simulink model "HDVSim_BEV_Truck"  (R2019b)
settings: Solver=ode3  StartTime=0.0  StopTime=inf  FixedStep=sample_time  MaxStep=0.1  RelTol=1e-3  EnableMultiTasking=on
model workspace (MAT data in the model file):
  Bat.SOC_start = 1
  Bat.Voltage = 800
  Bat.Useable_range = 0.8
  Bat.Charge_cycles = 3202.25561185
  Bat.Useable_capacity = 800
  Bat.Efficiency_power_electronics = 0.95
  Bat.Type = 1
  Electric_Truck = 1
  FuelCell.P_nom = 0
  Fueltype = 7
  Hybrid_Truck = 1
  IZ12 = 3600
  M_el = 1000
  SOC_T_EM_completely_available = 0.5
  SOC_addition = 0.4
  SOC_el = 0.8
  SOC_target = 0.85
  Sailing_without_drag_torque = 0
  TCO = TCO
  TCO.Ratio_Trailer_Truck = [1 1]
  TCO.Price_increase_repurchase = [3.5 3.5]
  TCO.Daily_working_time = 8
  TCO.Other_works_day = 0.5
  TCO.Gross_hourly_wage_driver = 13
  TCO.Operating_days_year = 240
  TCO.Annual_gross_wage_driver = 24960
  TCO.Personnel_factor = 1.3
  TCO.Annual_gross_wage_truck = 32448
  TCO.Social_costs_percent = 25.75
  TCO.Social_costs_EUR = 8355
  TCO.Back_up_driver = 0
  TCO.Fees_day = 12
  TCO.Fees_year = 2880
  TCO.Driver_costs_other = 0
  TCO.Driving_personnel_costs_total = 43683
  TCO.Diesel_price = 0.95
  TCO.Diesel_price_external = 1
  TCO.Adblue_price = 0.68
  TCO.CNG_price = 0.88
  TCO.LNG_price = 0.81
  TCO.Electricity_price = 0.12
  TCO.Hydrogen_price = 9
  TCO.Interest_current_asset = 8.4
  TCO.Interest_fixed_asset = 8.4
  TCO.Administrative_costs = 10.7
  TCO.Driving_distance = 0
  TCO.Ratio_toll_route = 75
  TCO.Loading_time_combination = 0.25
  TCO.Unloading_time_combination = 0.25
  TCO.Ratio_empty_trips = 0
  TCO.Operating_life = [6 12]
  TCO.Tire_mileage = [140000 170000]
  TCO.Ratio_inhouse_tanking_diesel = 75
  TCO.Lubricant_consumption = 1
  TCO.Adblue_consumption = 4
  TCO.Afa_time_dependent = [100 100]
  TCO.Afa_power_dependent = [0 0]
  TCO.Current_asset = [6000 1400]
  TCO.Insurance_vehicle = [0 0]
  TCO.Insurance_transport = 1000
  TCO.Communication = 600
  TCO.Repair_maintenance_care = [0.13 0.025]
  TCO.Current_assets_interest_bearing = 622
  TCO.Results = table
  TCO.Results.data = {{[]; []; []; []; []; []; []; []; []; []; []; []; []; []; []; []; []; []; []; []; []; []; []}, {[]; []; []; []; []; []; []; []; []; []; []; []; []; []; []; []; []; []; []; []; []; []; []}, {[]; []; []; []; []; []; []; []; []; []; []; []; []; []; []; []; []; []; []; []; []; []; []}, {'#cccccc'; '#9DFF00'; '#CEFF00'; '#FFFF00'; '#FFDF00'; '#FFB900'; '#FF9200'; '#FF5D00'; '#FF7F7F'; '#FF2900'; '#cccccc'; '#00FF85'; '#00FFC6'; '#00FFF2'; '#00FFFF'; '#00DBFF'; '#00B3FF'; '#0088FF'; '#cccccc'; '#B100FF'; '#FF00FF'; '#FF00C0'; '#FF0070'}, [0; 1; 1; 1; 1; 1; 1; 0; 1; 0; 0; 1; 1; 1; 1; 1; 1; 0; 0; 0; 1; 1; 0]}
  TCO.Results.ndims = 2
  TCO.Results.nrows = 23
  TCO.Results.rownames = {'Time_dependent_vehicle_costs'; 'Amortisation_time_dependent'; 'Current_assets_interest_bearing'; 'Fixed_assets_interest_bearing'; 'Taxes'; 'Insurance'; 'Communication'; 'Sum_vehicle_costs'; 'Driving_personnel_costs_total'; 'Sum_fix_costs'; 'Performance_related_vehicle_costs'; 'Amortisation_performance_related'; 'Fuel_costs'; 'Adblue_costs'; 'Repair_costs'; 'Lubricant_costs'; 'Tire_costs'; 'Sum_variable_costs'; 'Sum_costs'; 'Sum_fix_variable_costs'; 'Overhead_costs'; 'Toll_costs'; 'Total_costs'}
  TCO.Results.nvars = 5
  TCO.Results.varnames = {'Euro_Year', 'Euro_km', 'Percent', 'Cellcolor', 'Diagramm'}
  TCO.Results.props.useVariableNamesOriginal = 0
  TCO.Results.props.useDimensionNamesOriginal = 0
  TCO.Results.props.CustomProps = struct()
  TCO.Results.props.VariableCustomProps = struct()
  TCO.Results.props.versionSavedFrom = 4
  TCO.Results.props.minCompatibleVersion = 1
  TCO.Results.props.incompatibilityMsg = ''
  TCO.Results.props.VersionSavedFrom = 4
  TCO.Results.props.Description = ''
  TCO.Results.props.VariableNamesOriginal = {}
  TCO.Results.props.DimensionNames = {'Row', 'Variables'}
  TCO.Results.props.DimensionNamesOriginal = {}
  TCO.Results.props.UserData = []
  TCO.Results.props.VariableDescriptions = {}
  TCO.Results.props.VariableUnits = {}
  TCO.Results.props.VariableContinuity = {}
  TCO_Trailer = 1
  T_distance_LPS_down = 250
  T_distance_LPS_up = 250
  VSim.Display = 3
  VSim.Opt = 0
  VSim.v_t = [0 0 0 0 0 0 6.20410078977 13.0955619562 19.9830639689 26.8635610218 33.7348315113 40.5726013287 46.6919481688 50.4292373299 51.5990732528 55.4690950813 59.3274381556 63.1733217217 67.0059768235 70.7546293457 74.2808623311 77.6099839176 80.7667223894 83.4687787689 85.9844105019 87.7679000427 86.6050016922 86.7064046745 86.7114286994 86.7139311054 86.7163374998 86.7187109942 86.7210536154]
  Vehicle = 'empty'
  WPT.Voltage = 0
  WPT.P_max = 120
  WPT.expansion = 0.42
  WPT.eta = 0.92
  WPT.SOC_target = 1
  WPT.SOC_electric_only = 1
  acquisitionCosts = acquisitionCosts
  acquisitionCosts.KA_ZM = 361928.055317
  acquisitionCosts.KG = 3917.83103379
  acquisitionCosts.Getr_m = 135.266288088
  acquisitionCosts.KMot = 4672
  acquisitionCosts.KH = 179973.93
  acquisitionCosts.Hybrid = 1
  acquisitionCosts.Elektro = 1
  acquisitionCosts.Bat = 168200
  acquisitionCosts.Bat_type = 1
  acquisitionCosts.Bat_m = 5298.01324503
  acquisitionCosts.Bat_kWh = 800
  acquisitionCosts.Bat_VK_Pouch = 176
  acquisitionCosts.Bat_VK_Cyl = 210
  acquisitionCosts.Ratio_BEV2PHEV = 1
  acquisitionCosts.EM = 7717.5
  acquisitionCosts.EM_Type = 2
  acquisitionCosts.EM_P_max = 750
  acquisitionCosts.LE = 3375
  acquisitionCosts.FC = 0
  acquisitionCosts.P_FC = 0
  acquisitionCosts.KTFC_VK = 608
  acquisitionCosts.KA = 0
  acquisitionCosts.v_diesel = 0
  acquisitionCosts.v_cng = 0
  acquisitionCosts.v_lng = 0
  acquisitionCosts.m_h2 = 0
  acquisitionCosts.KT = 0
  acquisitionCosts.KTD = 0
  acquisitionCosts.KTCNG = 0
  acquisitionCosts.KTLNG = 0
  acquisitionCosts.KTFC = 0
  addition_for_critical_slope = 0.01
  ambient.gravity = 9.80665
  ambient.air_density = 1.1883
  ambient.friction_coeff = 0.8
  auxiliary_consumers.onBattery = 1
  auxiliary_consumers.power = 3500
  critical_altitude_difference = 50
  cycle.distance = [0 1 5 31 59 82 101 122 140 164 178 192 ... (10614 elements, 10614x1)]
  cycle.speed = [0 8.33333333333 8.33333333333 8.33333333333 8.33333333333 8.33333333333 8.33333333333 8.33333333333 8.33333333333 8.33333333333 8.33333333333 8.33333333333 ... (10614 elements, 10614x1)]
  cycle.slope = [0 0 0.0147 0.0305 0.0436 0.0483 0.0498 0.0479 0.0407 0.0324 0.0203 -0.0071 ... (10614 elements, 10614x1)]
  cycle.stop_time = [1 1 1 0 0 0 0 0 0 0 0 0 ... (10614 elements, 10614x1)]
  cycle.altitude = [0 0 0 0 0 0 0 0 0 0 0 0 ... (10614 elements, 10614x1)]
  cycle.stop_end = 15
  cycle.stop_start = 5
  cycle.speed_init = 1
  cycle.delta12 = [0 0 0 0 0 0 0 0 0 0 0 0 ... (10614 elements, 1x10614)]
  cycle.delta23 = [0 0 0 0 0 0 0 0 0 0 0 0 ... (10614 elements, 1x10614)]
  dcycle = 22
  distance_1_PPC = 175
  distance_2_PPC = 200
  distance_PPC_altitude_difference = 10000
  driver.controller_proportional_gain = 230000
  driver.controller_integral_gain = 3000
  driver.slew_rate_throttle_in = 2
  driver.slew_rate_throttle_out = -2
  driver.slew_rate_brake_in = 2
  driver.slew_rate_brake_out = -2
  em.P_max = 646.662302279
  em.M_max = 2040.65740249
  em.n_eck = 2525
  em.n_max = 4418
  em.speed = [0 27.786163522 55.572327044 83.358490566 111.144654088 138.93081761 166.716981132 194.503144654 222.289308176 250.075471698 277.86163522 305.647798742 ... (160 elements, 1x160)]
  em.trq = [2040.65740001 2040.65740051 2040.65740051 2040.65740211 2040.65740211 2040.65740249 2040.65740051 2040.65740051 2040.65740051 2040.65740051 2040.65740249 2040.65740051 ... (160 elements, 1x160)]
  em.Type = 2
  em.noEM = 2
  em.efficiency.characteristic_map = [0.001 0.001 0.001 0.001 0.001 0.001 0.001 0.001 0.001 0.001 0.001 0.001 ... (25600 elements, 160x160)]
  em.efficiency.speed = [0 27.786163522 55.572327044 83.358490566 111.144654088 138.93081761 166.716981132 194.503144654 222.289308176 250.075471698 277.86163522 305.647798742 ... (160 elements, 1x160)]
  em.efficiency.torque = [0 12.8343169968 25.6686339935 38.5029509903 51.3372679871 64.1715849838 77.0059019806 89.8402189773 102.674535974 115.508852971 128.343169968 141.177486964 ... (160 elements, 1x160)]
  em.shift_parameter.n_pref = 2398.75
  em.shift_parameter.n2 = 505
  em.shift_parameter.n6 = 3534.4
  em.fuel.co2_per_kwh = 504
  engine.M_max = 0
  engine.number = 4
  final_drive.ratio = 5
  final_drive.trq_eff = 0.98
  ifElectric = 1
  ifOptimized = 0
  look_ahead_PPC = 250
  max_distance = 100000
  name = 'HDVSim_BEV_Truck'
  preditiveCruiseControl = 0
  sample_time = 0.1
  tank.v_diesel = 0
  tank.v_lng = 0
  tank.v_cng = 0
  tank.m_h2 = 0
  tires.radius = 0.4465
  tires.roll_drag_coeff.total = 0.0043
  transmission.init_gear = 1
  transmission.shift_time = 1
  transmission.ratios = [1.7284 1]
  transmission.trq_eff = [0.96 0.99]
  transmission.lamda = [1.01169037498 1.00821410391]
  transmission.z = 2
  v_PPC_delta = 2.77777777778
  v_max_electrical_drive_only = 13.8888888889
  vehicle.long_truck = 0
  vehicle.payload = 19300
  vehicle.frontal_area = 10.2
  vehicle.air_drag_coeff = 0.53
  vehicle.Fx_max = 90221.18
  vehicle.F_brake_max = 309890.14
  vehicle.mass = 17056.2573109
  vehicleProperties = vehicleProperties
  vehicleProperties.CO2_EM_Range = 100
  vehicleProperties.a_0_80_Range = 54
  vehicleProperties.BOK_ak = 2.55
  vehicleProperties.BOK_Range = 4.65
  vehicleProperties.V_Rel_ak = 0.55
  vehicleProperties.V_Rel_Range = 0.35
  vehicleProperties.VWF_ak = 0.9
  vehicleProperties.VWF_Range = 7.2
  weights = weights
  weights.m_Gearbox = 135.266288088
  weights.m_Retarder = 82
  weights.m_Battery = 5298.01324503
  weights.m_EM = 833.333333333
  weights.m_PwrElectr = 69.4444444444
  weights.m_Charger = 15
  weights.m_Trailer = 5400
  weights.m_Total = 11656.2573109
  weights.m_Base = 5223.2
  weights.Electric = 1
  weights.Hybrid = 1
  weights.max_Payload = 23943.7426891
  weights.m_Max = 41000
  x = 1
values from neighbouring files (symbols this model uses):
  transmission = Transmission_gearing(15.86, 7, 0, 0, final_drive.ratio)    [Parameterizing.m]
undefined symbols (not defined in the file or in its folder): Ion, Lithium, prospective_cruise_control, Vorausschauender_Tempomat
libraries: simulink x21, powerlib x2, electricdrivelib x1
(part 1 of 3)
settings Model: Creator=Alexander Suessmann  LastModifiedBy=ubuntu
settings DataIOCC: SaveFormat=Array  SignalLoggingSaveFormat=ModelDataLogs  SaveOutput=off  SignalLogging=off  DSMLogging=off  ReturnWorkspaceOutputs=off  SignalLoggingName=datalog
settings OptimizationCC: ExpressionDepthLimit=2147483647  InitFltsAndDblsToZero=on  LifeSpan=inf
settings DebuggingCC: UnderspecifiedInitializationDetection=Classic  MergeDetectMultiDrivingBlocksExec=none  SolverPrmCheckMsg=warning  MultiTaskDSMMsg=warning  MultiTaskCondExecSysMsg=none  FcnCallInpInsideContextMsg=warning  AllowSymbolicDim=off  StateNameClashWarn=warning  SFUnexpectedBacktrackingDiag=warning  SFNoUnconditionalDefaultTransitionDiag=warning  SFExecutionAtInitializationDiag=none  UnderSpecifiedDimensionMsg=warning  ArithmeticOperatorsInVariantConditions=warning
settings HardwareCC: ProdBitPerPointer=32  ProdBitPerSizeT=32  ProdBitPerPtrDiffT=32  ProdLargestAtomicFloat=None  ProdIntDivRoundTo=Undefined  ProdEndianess=Unspecified  ProdWordSize=32  ProdHWDeviceType=32-bit Generic
settings ModelReferenceCC: PropagateSignalLabelsOutOfModel=off
settings SFSimCC: SimUseLocalCustomCode=off  CustomCodeUndefinedFunction=UseInterfaceOnly
settings RTWCC: RTWUseLocalCustomCode=off
settings CodeAppCC: StateflowObjectComments=on
settings GRTTargetCC: TargetLangStandard=C89/C90 (ANSI)  GeneratePreprocessorConditionals=Disable all  CombineOutputUpdateFcns=off  GRTInterface=on
settings ConfigComp: CovMetricSettings=dw  CovHtmlReporting=on  CovSaveCumulativeToWorkspaceVar=on  CovSaveSingleToWorkspaceVar=on  CovExternalEMLEnable=off  CovSFcnEnable=off
settings SimscapeCC: SimscapeNormalizeSystem=off

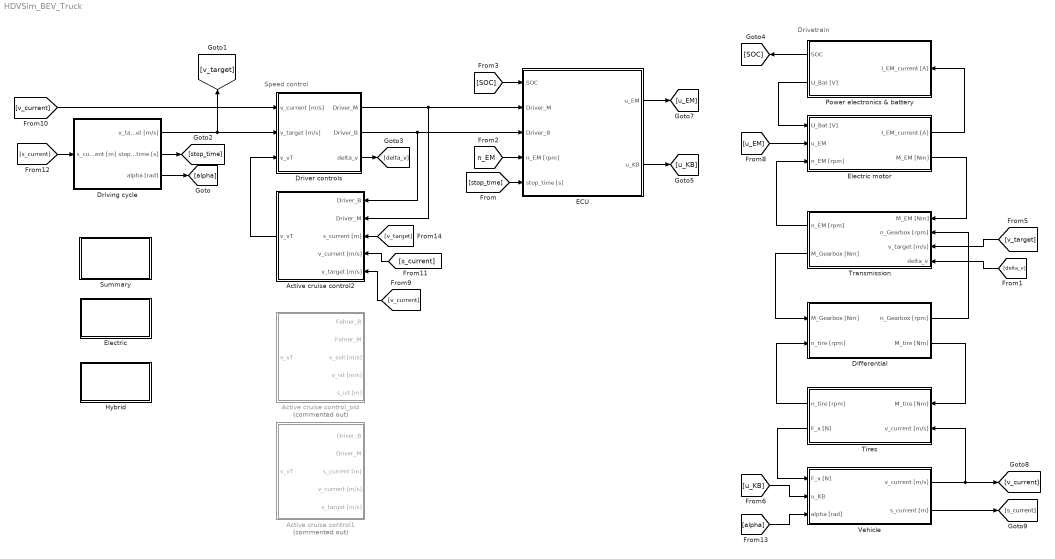
== system HDVSim_BEV_Truck ==
  note: Speed control
  note: Drivetrain
  Active cruise control1 : Subsystem  Commented=on
  Active cruise control2 : Subsystem
  Active cruise control_old : Subsystem  Commented=on
  Differential : Subsystem
  Driver controls : Subsystem
  Driving cycle : Subsystem
  ECU : Subsystem
  Electric : Subsystem
  Electric motor : Subsystem
  Hybrid : Subsystem
  Power electronics & battery : Subsystem
  Summary : Subsystem
  Tires : Subsystem
  Transmission : Subsystem
  Vehicle : Subsystem
  wires:
  Transmission/1(n_EM [rpm]) -> Electric motor/3(n_EM [rpm])
  Transmission/2(M_Gearbox [Nm]) -> Differential/1(M_Gearbox [Nm])
  Tires/1(n_tire [rpm]) -> Differential/2(n_tire [rpm])
  Differential/1(n_Gearbox [rpm]) -> Transmission/2(n_Gearbox [rpm])
  Differential/2(M_tire [Nm]) -> Tires/1(M_tire [Nm])
  Vehicle/1(v_current [m/s]) -> [v_current], Tires/2(v_current [m/s])
  Tires/2(F_x [N]) -> Vehicle/1(F_x [N])
  Driver controls/2(Driver_B) -> Active cruise control2/1(Driver_B), ECU/3(Driver_B)
  Electric motor/2(M_EM [Nm]) -> Transmission/1(M_EM [Nm])
  Electric motor/1(I_EM_current [A]) -> Power electronics & battery/1(I_EM_current [A])
  Power electronics & battery/2(U_Bat [V]) -> Electric motor/1(U_Bat [V])
  Active cruise control2/1(v_vT) -> Driver controls/3(v_vT)
  [n_EM] -> ECU/4(n_EM [rpm])
  Driving cycle/1(v_target [m/s]) -> [v_target], Driver controls/2(v_target [m/s])
  [v_current] -> Driver controls/1(v_current [m/s])
  [s_current] -> Driving cycle/1(s_current [m])
  Driver controls/1(Driver_M) -> Active cruise control2/2(Driver_M), ECU/2(Driver_M)
  Driving cycle/3(alpha [rad]) -> [alpha]
  Driving cycle/2(stop_time [s]) -> [stop_time]
  [stop_time] -> ECU/5(stop_time [s])
  Driver controls/3(delta_v) -> [delta_v]
  [SOC] -> ECU/1(SOC)
  [v_target] -> Active cruise control2/3(s_current [m])
  [s_current] -> Active cruise control2/4(v_current [m/s])
  [v_current] -> Active cruise control2/5(v_target [m/s])
  ECU/1(u_EM) -> [u_EM]
  ECU/2(u_KB) -> [u_KB]
  Power electronics & battery/1(SOC) -> [SOC]
  [u_EM] -> Electric motor/2(u_EM)
  [v_target] -> Transmission/3(v_target [m/s])
  [delta_v] -> Transmission/4(delta_v)
  Vehicle/2(s_current [m]) -> [s_current]
  [u_KB] -> Vehicle/2(u_KB)
  [alpha] -> Vehicle/3(alpha [rad])

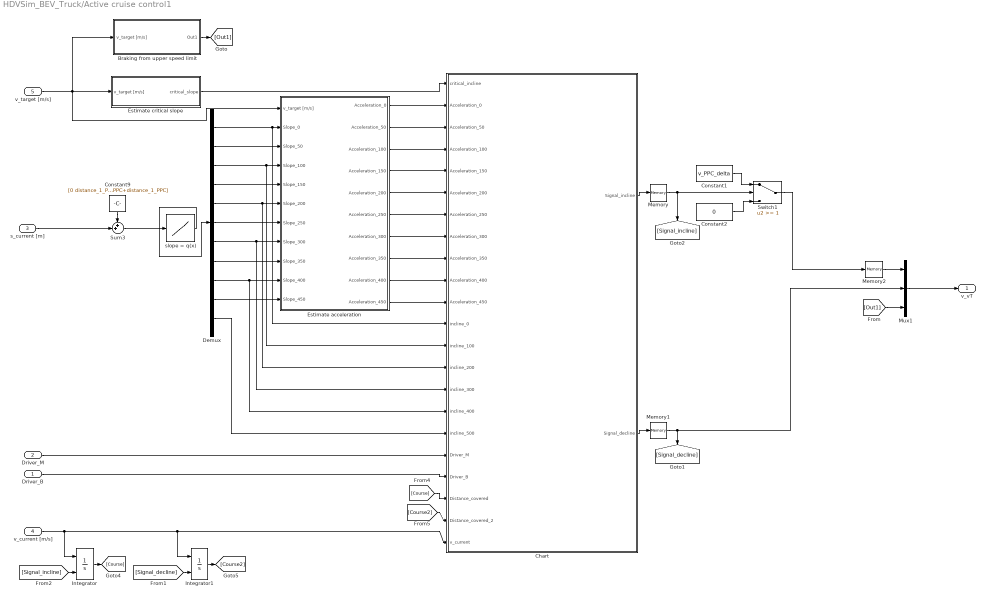
== system HDVSim_BEV_Truck/Active cruise control1 ==
  Driver_B : Inport
  Driver_M : Inport  Port=2
  s_current [m] : Inport  Port=3
  v_current [m/s] : Inport  Port=4
  v_target [m/s] : Inport  Port=5
  Braking from upper speed limit : Subsystem
  Chart : Stateflow chart  TreatAsAtomicUnit=on
  Constant1 : Constant  Value=v_PPC_delta
  Constant2 : Constant  Value=0
  Constant9 : Constant  Value=[0 distance_1_PPC/5 2*distance_1_PPC/5 3*distance_1_PPC/5 4*distance_1_PPC/5 distance_1_PPC 6*distance_1_PPC/5 7*distance_1_PPC/5 8*distance_1_PPC/5 9*distance_1_PPC/5 10*distance_1_PPC/5 look_ahead_PPC look_ahead_PPC+distance_1_PPC]
  Demux : Demux  Outputs=11
  Estimate acceleration : Subsystem
  Estimate critical slope : Subsystem
  Integrator : Integrator  ExternalReset=rising
  Integrator1 : Integrator  ExternalReset=rising
  Memory : Memory
  Memory1 : Memory
  Memory2 : Memory
  Mux1 : Mux  Inputs=3
  Sum3 : Sum  Inputs=++|
  Switch1 : Switch  Threshold=1
  slope = q(x) : Lookup  InputValues=cycle.distance  Table=cycle.slope  LookUpMeth=Interpolation-Use End Values
  v_vT : Outport  VectorParamsAs1DForOutWhenUnconnected=off
  wires:
  slope = q(x)/1 -> Demux/1
  Demux/1 -> Chart/12(incline_0), Estimate acceleration/2(Slope_0)
  Estimate critical slope/1(critical_slope) -> Chart/1(critical_incline)
  Chart/1(Signal_incline) -> Memory/1
  v_current [m/s]/1 -> Integrator/1, Integrator1/1, Chart/22(v_current)
  Memory/1 -> [Signal_incline], Switch1/2
  Mux1/1 -> v_vT/1
  Constant9/1 -> Sum3/1
  Sum3/1 -> slope = q(x)/1
  Estimate acceleration/1(Acceleration_0) -> Chart/2(Acceleration_0)
  Estimate acceleration/2(Acceleration_50) -> Chart/3(Acceleration_50)
  Estimate acceleration/3(Acceleration_100) -> Chart/4(Acceleration_100)
  Estimate acceleration/4(Acceleration_150) -> Chart/5(Acceleration_150)
  Estimate acceleration/5(Acceleration_200) -> Chart/6(Acceleration_200)
  Estimate acceleration/6(Acceleration_250) -> Chart/7(Acceleration_250)
  Estimate acceleration/7(Acceleration_300) -> Chart/8(Acceleration_300)
  Estimate acceleration/8(Acceleration_350) -> Chart/9(Acceleration_350)
  Chart/2(Signal_decline) -> Memory1/1
  Memory1/1 -> Mux1/2, [Signal_decline]
  Driver_B/1 -> Chart/19(Driver_B)
  Estimate acceleration/9(Acceleration_400) -> Chart/10(Acceleration_400)
  Estimate acceleration/10(Acceleration_450) -> Chart/11(Acceleration_450)
  Driver_M/1 -> Chart/18(Driver_M)
  Demux/2 -> Estimate acceleration/3(Slope_50)
  Demux/3 -> Chart/13(incline_100), Estimate acceleration/4(Slope_100)
  Demux/4 -> Estimate acceleration/5(Slope_150)
  Demux/5 -> Chart/14(incline_200), Estimate acceleration/6(Slope_200)
  Demux/6 -> Estimate acceleration/7("Slope_250 ")
  Demux/7 -> Chart/15(incline_300), Estimate acceleration/8(Slope_300)
  Demux/8 -> Estimate acceleration/9(Slope_350)
  Demux/9 -> Chart/16(incline_400), Estimate acceleration/10(Slope_400)
  Demux/10 -> Estimate acceleration/11(Slope_450)
  v_target [m/s]/1 -> Braking from upper speed limit/1(v_target [m/s]), Estimate acceleration/1(v_target [m/s]), Estimate critical slope/1(v_target [m/s])
  Memory2/1 -> Mux1/1
  Constant1/1 -> Switch1/1
  Constant2/1 -> Switch1/3
  Demux/11 -> Chart/17(incline_500)
  Switch1/1 -> Memory2/1
  s_current [m]/1 -> Sum3/2
  [Signal_decline] -> Integrator1/2
  Integrator1/1 -> [Course2]
  Integrator/1 -> [Course]
  [Signal_incline] -> Integrator/2
  [Course] -> Chart/20(Distance_covered)
  [Course2] -> Chart/21(Distance_covered_2)
  Braking from upper speed limit/1(Out1) -> [Out1]
  [Out1] -> Mux1/3

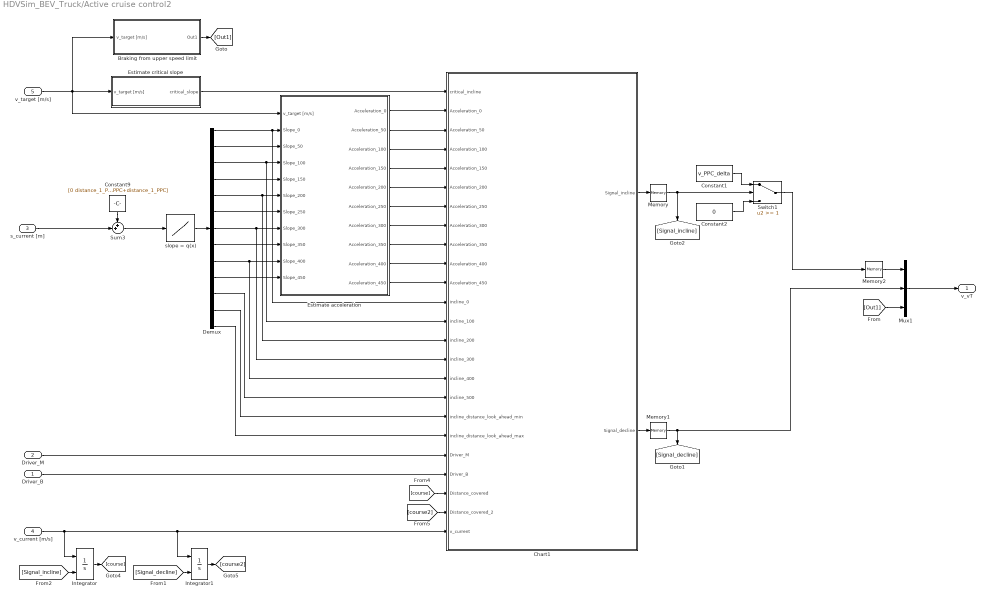
== system HDVSim_BEV_Truck/Active cruise control2 ==
  Driver_B : Inport
  Driver_M : Inport  Port=2
  s_current [m] : Inport  Port=3
  v_current [m/s] : Inport  Port=4
  v_target [m/s] : Inport  Port=5
  Braking from upper speed limit : Subsystem
  Chart1 : Stateflow chart  TreatAsAtomicUnit=on
  Constant1 : Constant  Value=v_PPC_delta
  Constant2 : Constant  Value=0
  Constant9 : Constant  Value=[0 distance_1_PPC/5 2*distance_1_PPC/5 3*distance_1_PPC/5 4*distance_1_PPC/5 distance_1_PPC 6*distance_1_PPC/5 7*distance_1_PPC/5 8*distance_1_PPC/5 9*distance_1_PPC/5 10*distance_1_PPC/5 look_ahead_PPC look_ahead_PPC+distance_1_PPC]
  Demux : Demux  Outputs=13
  Estimate acceleration : Subsystem
  Estimate critical slope : Subsystem
  Integrator : Integrator  ExternalReset=rising
  Integrator1 : Integrator  ExternalReset=rising
  Memory : Memory
  Memory1 : Memory
  Memory2 : Memory
  Mux1 : Mux  Inputs=3
  Sum3 : Sum  Inputs=++|
  Switch1 : Switch  Threshold=1
  slope = q(x) : Lookup  InputValues=cycle.distance  Table=cycle.slope  LookUpMeth=Interpolation-Use End Values
  v_vT : Outport  VectorParamsAs1DForOutWhenUnconnected=off
  wires:
  slope = q(x)/1 -> Demux/1
  Demux/1 -> Chart1/12(incline_0), Estimate acceleration/2(Slope_0)
  Estimate critical slope/1(critical_slope) -> Chart1/1(critical_incline)
  Chart1/1(Signal_incline) -> Memory/1
  v_current [m/s]/1 -> Integrator/1, Chart1/24(v_current), Integrator1/1
  Memory/1 -> [Signal_incline], Switch1/2
  Mux1/1 -> v_vT/1
  Constant9/1 -> Sum3/1
  Sum3/1 -> slope = q(x)/1
  Estimate acceleration/1(Acceleration_0) -> Chart1/2(Acceleration_0)
  Estimate acceleration/2(Acceleration_50) -> Chart1/3(Acceleration_50)
  Estimate acceleration/3(Acceleration_100) -> Chart1/4(Acceleration_100)
  Estimate acceleration/4(Acceleration_150) -> Chart1/5(Acceleration_150)
  Estimate acceleration/5(Acceleration_200) -> Chart1/6(Acceleration_200)
  Estimate acceleration/6(Acceleration_250) -> Chart1/7(Acceleration_250)
  Estimate acceleration/7(Acceleration_300) -> Chart1/8(Acceleration_300)
  Estimate acceleration/8(Acceleration_350) -> Chart1/9(Acceleration_350)
  Chart1/2(Signal_decline) -> Memory1/1
  Memory1/1 -> Mux1/2, [Signal_decline]
  Driver_B/1 -> Chart1/21(Driver_B)
  Estimate acceleration/9(Acceleration_400) -> Chart1/10(Acceleration_400)
  Estimate acceleration/10(Acceleration_450) -> Chart1/11(Acceleration_450)
  Driver_M/1 -> Chart1/20(Driver_M)
  Demux/2 -> Estimate acceleration/3(Slope_50)
  Demux/3 -> Chart1/13(incline_100), Estimate acceleration/4(Slope_100)
  Demux/4 -> Estimate acceleration/5(Slope_150)
  Demux/5 -> Chart1/14(incline_200), Estimate acceleration/6(Slope_200)
  Demux/6 -> Estimate acceleration/7("Slope_250 ")
  Demux/7 -> Chart1/15(incline_300), Estimate acceleration/8(Slope_300)
  Demux/8 -> Estimate acceleration/9(Slope_350)
  Demux/9 -> Chart1/16(incline_400), Estimate acceleration/10(Slope_400)
  Demux/10 -> Estimate acceleration/11(Slope_450)
  Demux/12 -> Chart1/18(incline_distance_look_ahead_min)
  Demux/13 -> Chart1/19(incline_distance_look_ahead_max)
  v_target [m/s]/1 -> Braking from upper speed limit/1(v_target [m/s]), Estimate acceleration/1(v_target [m/s]), Estimate critical slope/1(v_target [m/s])
  Memory2/1 -> Mux1/1
  Constant1/1 -> Switch1/1
  Constant2/1 -> Switch1/3
  Demux/11 -> Chart1/17(incline_500)
  Switch1/1 -> Memory2/1
  s_current [m]/1 -> Sum3/2
  [Signal_decline] -> Integrator1/2
  Integrator1/1 -> [course2]
  Integrator/1 -> [course]
  [Signal_incline] -> Integrator/2
  [course] -> Chart1/22(Distance_covered)
  [course2] -> Chart1/23(Distance_covered_2)
  Braking from upper speed limit/1(Out1) -> [Out1]
  [Out1] -> Mux1/3

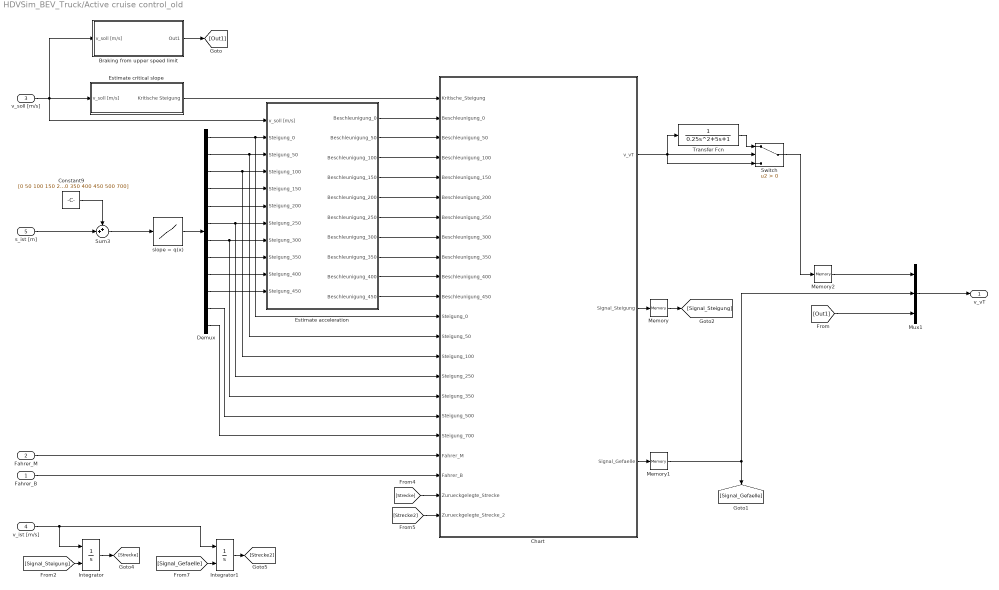
== system HDVSim_BEV_Truck/Active cruise control_old ==
  Fahrer_B : Inport
  Fahrer_M : Inport  Port=2
  v_soll [m/s] : Inport  Port=3
  v_ist [m/s] : Inport  Port=4
  s_ist [m] : Inport  Port=5
  Braking from upper speed limit : Subsystem
  Chart : Stateflow chart  TreatAsAtomicUnit=on
  Constant9 : Constant  Value=[0 50 100 150 200 250 300 350 400 450 500 700]
  Demux : Demux  Outputs=12
  Estimate acceleration : Subsystem
  Estimate critical slope : Subsystem
  Integrator : Integrator  ExternalReset=rising
  Integrator1 : Integrator  ExternalReset=rising
  Memory : Memory
  Memory1 : Memory
  Memory2 : Memory
  Mux1 : Mux  Inputs=3
  Sum3 : Sum  Inputs=++|
  Switch : Switch  Criteria=u2 > Threshold
  Transfer Fcn : TransferFcn  Denominator=[0.25 5 1]
  slope = q(x) : Lookup  InputValues=cycle.distance  Table=cycle.slope  LookUpMeth=Interpolation-Use End Values
  v_vT : Outport  VectorParamsAs1DForOutWhenUnconnected=off
  wires:
  slope = q(x)/1 -> Demux/1
  Demux/1 -> Estimate acceleration/2(Steigung_0), Chart/12(Steigung_0)
  Estimate critical slope/1(Kritische Steigung) -> Chart/1(Kritische_Steigung)
  Chart/2(Signal_Steigung) -> Memory/1
  Mux1/1 -> v_vT/1
  Constant9/1 -> Sum3/1
  s_ist [m]/1 -> Sum3/2
  Sum3/1 -> slope = q(x)/1
  Estimate acceleration/1(Beschleunigung_0) -> Chart/2(Beschleunigung_0)
  Estimate acceleration/2(Beschleunigung_50) -> Chart/3(Beschleunigung_50)
  Estimate acceleration/3(Beschleunigung_100) -> Chart/4(Beschleunigung_100)
  Estimate acceleration/4(Beschleunigung_150) -> Chart/5(Beschleunigung_150)
  Estimate acceleration/5(Beschleunigung_200) -> Chart/6(Beschleunigung_200)
  Estimate acceleration/6(Beschleunigung_250) -> Chart/7(Beschleunigung_250)
  Estimate acceleration/7(Beschleunigung_300) -> Chart/8(Beschleunigung_300)
  Estimate acceleration/8(Beschleunigung_350) -> Chart/9(Beschleunigung_350)
  Chart/3(Signal_Gefaelle) -> Memory1/1
  Memory1/1 -> [Signal_Gefaelle], Mux1/2
  Fahrer_B/1 -> Chart/20(Fahrer_B)
  Estimate acceleration/9(Beschleunigung_400) -> Chart/10(Beschleunigung_400)
  Estimate acceleration/10(Beschleunigung_450) -> Chart/11(Beschleunigung_450)
  Fahrer_M/1 -> Chart/19(Fahrer_M)
  Demux/2 -> Estimate acceleration/3(Steigung_50), Chart/13(Steigung_50)
  Demux/3 -> Estimate acceleration/4(Steigung_100), Chart/14(Steigung_100)
  Demux/4 -> Estimate acceleration/5(Steigung_150)
  Demux/5 -> Estimate acceleration/6(Steigung_200)
  Demux/6 -> Estimate acceleration/7("Steigung_250 "), Chart/15(Steigung_250)
  Demux/7 -> Estimate acceleration/8(Steigung_300), Chart/16(Steigung_350)
  Demux/8 -> Estimate acceleration/9(Steigung_350)
  Demux/9 -> Estimate acceleration/10(Steigung_400)
  Demux/10 -> Estimate acceleration/11(Steigung_450)
  Demux/11 -> Chart/17(Steigung_500)
  Demux/12 -> Chart/18(Steigung_700)
  v_soll [m/s]/1 -> Braking from upper speed limit/1(v_soll [m/s]), Estimate acceleration/1(v_soll [m/s]), Estimate critical slope/1(v_soll [m/s])
  Memory2/1 -> Mux1/1
  Switch/1 -> Memory2/1
  Chart/1(v_vT) -> Switch/2, Switch/3, Transfer Fcn/1
  Transfer Fcn/1 -> Switch/1
  Braking from upper speed limit/1(Out1) -> [Out1]
  [Out1] -> Mux1/3
  Memory/1 -> [Signal_Steigung]
  [Signal_Gefaelle] -> Integrator1/2
  Integrator1/1 -> [Strecke2]
  v_ist [m/s]/1 -> Integrator1/1, Integrator/1
  [Signal_Steigung] -> Integrator/2
  Integrator/1 -> [Strecke]
  [Strecke] -> Chart/21(Zurueckgelegte_Strecke)
  [Strecke2] -> Chart/22(Zurueckgelegte_Strecke_2)

== system HDVSim_BEV_Truck/Differential ==
  note: Effective wheel torque
  M_Gearbox [Nm] : Inport
  n_tire [rpm] : Inport  Port=2
  Differential efficiency : Constant  Value=final_drive.trq_eff
  Differential gear ratio : Constant  Value=final_drive.ratio
  Gain : Gain  Commented=on  Gain=2*pi/(60 * 1000)
  M' = M*i*eta : Product  Inputs=***
  Product : Product  Inputs=/  RndMeth=Zero
  Scope1 : Scope  Commented=on
  Switch : Switch  ZeroCross=off
  n' *i = n : Product  RndMeth=Zero
  n' *i = n1 : Product  Commented=on  RndMeth=Zero
  n_Gearbox [rpm] : Outport  VectorParamsAs1DForOutWhenUnconnected=off
  M_tire [Nm] : Outport  Port=2  VectorParamsAs1DForOutWhenUnconnected=off
  wires:
  M_Gearbox [Nm]/1 -> M' = M*i*eta/1, Switch/2
  Differential gear ratio/1 -> n' *i = n/1, M' = M*i*eta/3
  n' *i = n/1 -> n_Gearbox [rpm]/1
  Differential efficiency/1 -> Product/1, Switch/1
  Product/1 -> Switch/3
  Switch/1 -> M' = M*i*eta/2
  n_tire [rpm]/1 -> n' *i = n1/1, n' *i = n/2
  M' = M*i*eta/1 -> n' *i = n1/2, M_tire [Nm]/1
  n' *i = n1/1 -> Gain/1
  Gain/1 -> Scope1/1

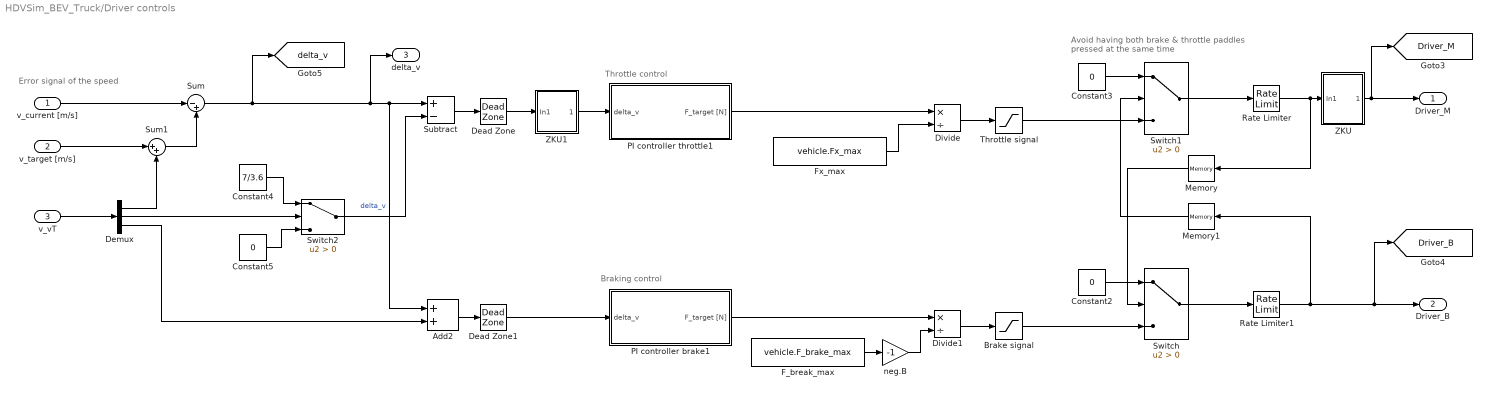
== system HDVSim_BEV_Truck/Driver controls ==
  note: Error signal of the speed
  note: Throttle control
  note: Braking control
  note: Avoid having both brake & throttle
      | paddles pressed at the same time
  v_current [m/s] : Inport
  v_target [m/s] : Inport  Port=2
  v_vT : Inport  Port=3
  Add2 : Sum
  Brake signal : Saturate  UpperLimit=1  LowerLimit=0  ZeroCross=off
  Constant2 : Constant  Value=0
  Constant3 : Constant  Value=0
  Constant4 : Constant  Value=7/3.6
  Constant5 : Constant  Value=0
  Dead Zone : DeadZone  LowerValue=-0.1/3.6  UpperValue=0.1/3.6  ZeroCross=off  SaturateOnIntegerOverflow=on
  Dead Zone1 : DeadZone  LowerValue=-0.1/3.6  UpperValue=0  ZeroCross=off  SaturateOnIntegerOverflow=on
  Demux : Demux  Outputs=3
  Divide : Product  Inputs=*/
  Divide1 : Product  Inputs=*/
  F_break_max : Constant  Value=vehicle.F_brake_max
  Fx_max : Constant  Value=vehicle.Fx_max
  Memory : Memory
  Memory1 : Memory
  PI controller brake1 : Subsystem
  PI controller throttle1 : Subsystem
  Rate Limiter : RateLimiter  RisingSlewLimit=driver.slew_rate_throttle_in  FallingSlewLimit=driver.slew_rate_throttle_out  SampleTimeMode=inherited
  Rate Limiter1 : RateLimiter  RisingSlewLimit=driver.slew_rate_brake_in*100  FallingSlewLimit=driver.slew_rate_brake_out*100  SampleTimeMode=inherited
  Subtract : Sum  Inputs=+-
  Sum : Sum  Inputs=|-+
  Sum1 : Sum  Inputs=|++
  Switch : Switch  Criteria=u2 > Threshold
  Switch1 : Switch  Criteria=u2 > Threshold
  Switch2 : Switch  Criteria=u2 > Threshold
  Throttle signal : Saturate  UpperLimit=1  LowerLimit=0  ZeroCross=off
  ZKU : Subsystem
  ZKU1 : Subsystem
  neg.B : Gain  Gain=-1
  Driver_M : Outport  VectorParamsAs1DForOutWhenUnconnected=off
  Driver_B : Outport  Port=2  VectorParamsAs1DForOutWhenUnconnected=off
  delta_v : Outport  Port=3  VectorParamsAs1DForOutWhenUnconnected=off
  tag scope: Driver_B=global, Driver_M=global, delta_v=global
  wires:
  Fx_max/1 -> Divide/2
  neg.B/1 -> Divide1/2
  Divide1/1 -> Brake signal/1
  Divide/1 -> Throttle signal/1
  F_break_max/1 -> neg.B/1
  Switch/1 -> Rate Limiter1/1
  Brake signal/1 -> Switch/3
  Constant2/1 -> Switch/1
  Switch1/1 -> Rate Limiter/1
  Throttle signal/1 -> Switch1/3
  Rate Limiter1/1 -> Memory1/1, [Driver_B], Driver_B/1
  Rate Limiter/1 -> ZKU/1(In1), Memory/1
  Constant3/1 -> Switch1/1
  PI controller throttle1/1(F_target [N]) -> Divide/1
  PI controller brake1/1(F_target [N]) -> Divide1/1
  ZKU/1(Out1) -> [Driver_M], Driver_M/1
  Memory/1 -> Switch/2
  Memory1/1 -> Switch1/2
  Sum1/1 -> Sum/2
  v_current [m/s]/1 -> Sum/1
  Sum/1 -> [delta_v], delta_v/1, Add2/1, Subtract/1  "delta_v"
  Dead Zone/1 -> ZKU1/1(In1)
  Dead Zone1/1 -> PI controller brake1/1(delta_v)
  ZKU1/1(Out1) -> PI controller throttle1/1(delta_v)
  v_vT/1 -> Demux/1
  Switch2/1 -> Subtract/2
  Demux/2 -> Switch2/2
  Constant4/1 -> Switch2/1
  Constant5/1 -> Switch2/3
  Subtract/1 -> Dead Zone/1
  Demux/1 -> Sum1/2
  v_target [m/s]/1 -> Sum1/1
  Demux/3 -> Add2/2
  Add2/1 -> Dead Zone1/1

== system HDVSim_BEV_Truck/Driving cycle ==
  note: Lookup tables
  s_current [m] : Inport
  Clock : Clock
  Compare To Constant : simulink/Logic and Bit Operations/Compare To Constant  relop=>=  const=max_distance  OutDataTypeStr=boolean
  Constant : Constant  Value=0
  Holding time at the beginning : Subsystem
  Holding time at the end : Subsystem
  Significant speed deviation : Subsystem
  Slope-> angle : Trigonometry  Operator=atan
  Stop Simulation : Stop
  Stop Simulation 2 : Stop
  Switch : Switch  Criteria=u2 > Threshold
  Terminator : Terminator
  altitude : Lookup_n-D  NumberOfTableDimensions=1  BreakpointsForDimension1=cycle.distance  Table=cycle.altitude  InterpMethod=Flat  RndMeth=Simplest  InputSameDT=on
  slope : Lookup_n-D  NumberOfTableDimensions=1  BreakpointsForDimension1=cycle.distance  Table=cycle.slope  InterpMethod=Flat  RndMeth=Simplest  InputSameDT=on
  speed : Lookup_n-D  NumberOfTableDimensions=1  BreakpointsForDimension1=cycle.distance  Table=cycle.speed  InterpMethod=Flat  RndMeth=Simplest  InputSameDT=on
  stop_time : Lookup_n-D  NumberOfTableDimensions=1  BreakpointsForDimension1=cycle.distance  Table=cycle.stop_time  InterpMethod=Flat  RndMeth=Simplest  InputSameDT=on
  v_target [m/s] : Outport  VectorParamsAs1DForOutWhenUnconnected=off
  stop_time [s] : Outport  Port=2  VectorParamsAs1DForOutWhenUnconnected=off
  alpha [rad] : Outport  Port=3  VectorParamsAs1DForOutWhenUnconnected=off
  tag scope: altitude=global, slope_q=global, v_target_dc=global
  wires:
  slope/1 -> Slope-> angle/1, [slope_q]
  Slope-> angle/1 -> alpha [rad]/1
  Compare To Constant/1 -> Holding time at the end/1(In1)
  Clock/1 -> Terminator/1  "duration"
  Switch/1 -> [v_target_dc], v_target [m/s]/1
  s_current [m]/1 -> slope/1, Significant speed deviation/1(In1), Compare To Constant/1, altitude/1, speed/1, stop_time/1
  stop_time/1 -> stop_time [s]/1, Switch/2
  speed/1 -> Holding time at the beginning/1(In1)
  Holding time at the end/1(Out1) -> Stop Simulation/1
  Holding time at the beginning/1(Out1) -> Switch/3
  Constant/1 -> Switch/1
  altitude/1 -> [altitude]
  Significant speed deviation/1(Out1) -> Stop Simulation 2/1

== system HDVSim_BEV_Truck/ECU ==
  SOC : Inport
  Driver_M : Inport  Port=2
  Driver_B : Inport  Port=3
  n_EM [rpm] : Inport  Port=4
  stop_time [s] : Inport  Port=5
  Approach to stop : Subsystem
  Calculations for braking : Subsystem
  Calculations for throttle : Subsystem
  Chart : Stateflow chart  TreatAsAtomicUnit=on
  Saturation : Saturate  UpperLimit=1  LowerLimit=-1
  Saturation1 : Saturate  UpperLimit=vehicle.Fx_max  LowerLimit=-vehicle.Fx_max
  Saturation2 : Saturate  UpperLimit=1  LowerLimit=0
  Scope : Scope  NumInputPorts=6
  Sum : Sum  Inputs=++|
  Sum1 : Sum  Inputs=++|
  u_EM : Outport  VectorParamsAs1DForOutWhenUnconnected=off
  u_KB : Outport  Port=2  VectorParamsAs1DForOutWhenUnconnected=off
  tag scope: REKUP=global
  wires:
  Chart/1(u_EM) -> Saturation/1
  Chart/2(u_KB) -> Saturation2/1
  Sum1/1 -> Chart/2(Driver_B), Calculations for braking/2(Driver_B)
  Sum/1 -> Chart/1(Driver_M), Calculations for throttle/1(Driver_M)
  Calculations for braking/2(F_brake_elec_max [N]) -> Saturation1/1
  Calculations for braking/1(F_brake_required [N]) -> Chart/6(F_brake_required)
  SOC/1 -> Chart/3(SOC), Calculations for throttle/2(SOC)
  Calculations for throttle/2(M_Required [Nm]) -> Chart/5(M_required)
  Saturation2/1 -> u_KB/1, Scope/2  "u_KB"
  Chart/3(ROLL) -> Scope/3  "ROLL"
  Chart/4(REKUP) -> [REKUP], Scope/4  "REKUP"
  [slope_q] -> Scope/5  "Slope"
  Calculations for throttle/1(M_EM_max [Nm]) -> Chart/4(M_EM_max), Calculations for braking/1(M_EM_max [Nm])
  [SOC] -> Scope/6  "SOC"
  Saturation/1 -> u_EM/1, Scope/1  "u_EM"
  stop_time [s]/1 -> Approach to stop/1(stop_time [s])
  Approach to stop/2(Driver_B) -> Sum1/1
  Approach to stop/1(Driver_M) -> Sum/1
  Driver_M/1 -> Sum/2
  Driver_B/1 -> Sum1/2
  n_EM [rpm]/1 -> Calculations for throttle/3(n_EM [rpm])
  [gear] -> Calculations for braking/3(Gear)
  Saturation1/1 -> Chart/7(F_brake_el_max)

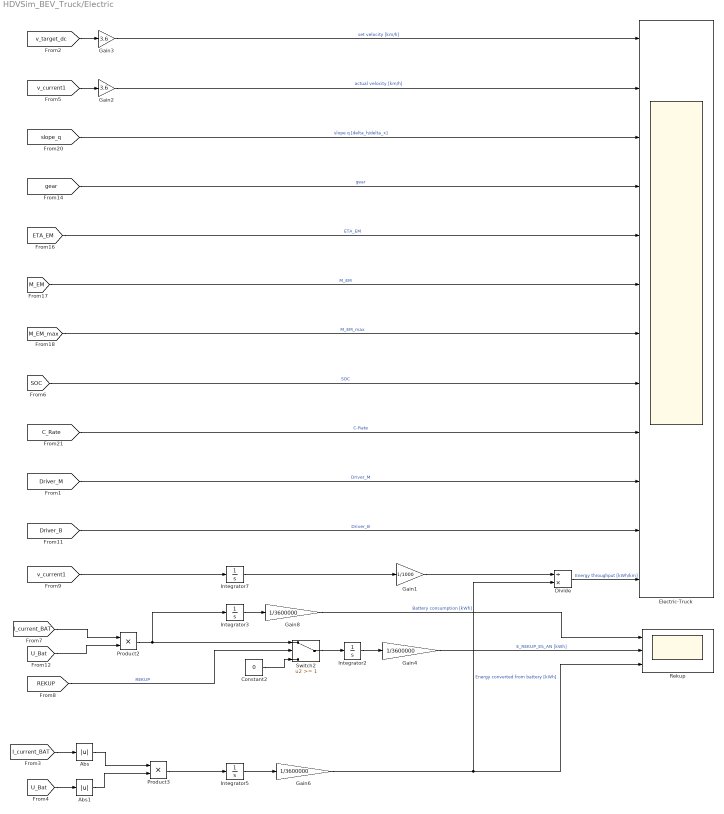
== system HDVSim_BEV_Truck/Electric ==
  Abs : Abs
  Abs1 : Abs
  Constant2 : Constant  Value=0
  Divide : Product  Inputs=/*
  Electric-Truck : Scope  NumInputPorts=12
  Gain1 : Gain  Gain=1/1000
  Gain2 : Gain  Gain=3.6
  Gain3 : Gain  Gain=3.6
  Gain4 : Gain  Gain=1/3600000
  Gain6 : Gain  Gain=1/3600000
  Gain8 : Gain  Gain=1/3600000
  Integrator2 : Integrator
  Integrator3 : Integrator
  Integrator5 : Integrator
  Integrator7 : Integrator  InitialCondition=0.00000001
  Product2 : Product
  Product3 : Product
  Rekup : Scope  NumInputPorts=3
  Switch2 : Switch  Threshold=1
  wires:
  [v_target_dc] -> Gain3/1
  Gain3/1 -> Electric-Truck/1  "set velocity [km/h]"
  [v_current1] -> Gain2/1
  Gain2/1 -> Electric-Truck/2  "actual velocity [km/h]"
  Gain4/1 -> Rekup/2  "E_REKUP_ES_AN [kWh]"
  Constant2/1 -> Switch2/3
  Integrator2/1 -> Gain4/1
  Switch2/1 -> Integrator2/1
  [REKUP] -> Switch2/2  "REKUP"
  [U_Bat] -> Product2/2
  [I_current_BAT] -> Product2/1
  [gear] -> Electric-Truck/4  "gear"
  [ETA_EM] -> Electric-Truck/5  "ETA_EM"
  [M_EM] -> Electric-Truck/6  "M_EM"
  [M_EM_max] -> Electric-Truck/7  "M_EM_max"
  [SOC] -> Electric-Truck/8  "SOC"
  Product2/1 -> Switch2/1, Integrator3/1
  Gain8/1 -> Rekup/1  "Battery consumption [kWh]"
  Integrator3/1 -> Gain8/1
  [U_Bat] -> Abs1/1
  [I_current_BAT] -> Abs/1
  Product3/1 -> Integrator5/1
  Integrator5/1 -> Gain6/1
  Abs/1 -> Product3/1
  Abs1/1 -> Product3/2
  [slope_q] -> Electric-Truck/3  "slope q [delta_h/delta_x]"
  [C_Rate] -> Electric-Truck/9  "C-Rate"
  [Driver_M] -> Electric-Truck/10  "Driver_M"
  [Driver_B] -> Electric-Truck/11  "Driver_B"
  Gain6/1 -> Divide/2, Rekup/3  "Energy converted from battery [kWh]"
  [v_current1] -> Integrator7/1
  Integrator7/1 -> Gain1/1
  Divide/1 -> Electric-Truck/12  "Energy throughput [kWh/km]"
  Gain1/1 -> Divide/1

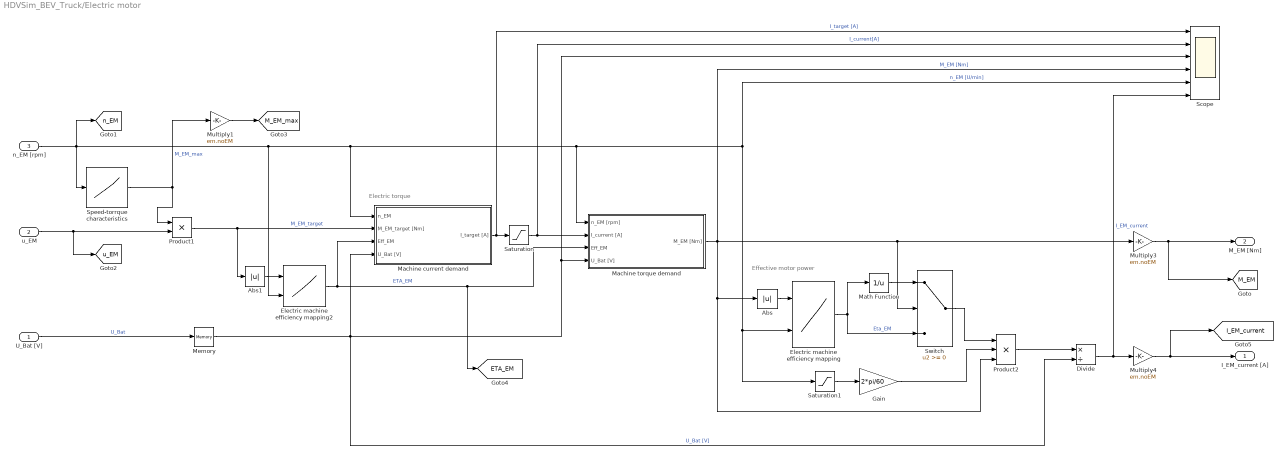
== system HDVSim_BEV_Truck/Electric motor ==
  note: Electric torque
  note: Effective motor power
  U_Bat [V] : Inport
  u_EM : Inport  Port=2
  n_EM [rpm] : Inport  Port=3
  Abs : Abs
  Abs1 : Abs
  Divide : Product  Inputs=*/
  Electric machine efficiency mapping : Lookup_n-D  BreakpointsForDimension1=em.efficiency.torque  BreakpointsForDimension2=em. efficiency.speed  BeginIndexSearchUsingPreviousIndexResult=on  Table=em.efficiency.characteristic_map  ExtrapMethod=Clip  UseLastTableValue=on  InternalRulePriority=Speed  RndMeth=Simplest  InputSameDT=on
  Electric machine efficiency mapping2 : Lookup_n-D  BreakpointsForDimension1=em.efficiency.torque  BreakpointsForDimension2=em.efficiency.speed  BeginIndexSearchUsingPreviousIndexResult=on  Table=em.efficiency.characteristic_map  ExtrapMethod=Clip  UseLastTableValue=on  InternalRulePriority=Speed  RndMeth=Simplest  InputSameDT=on
  Gain : Gain  Gain=2*pi/60
  Machine current demand : Subsystem
  Machine torque demand : Subsystem
  Math Function : Math  Operator=reciprocal  SaturateOnIntegerOverflow=on
  Memory : Memory  InitialCondition=1.0943*Bat.Voltage
  Multiply1 : Gain  Gain=em.noEM
  Multiply3 : Gain  Gain=em.noEM
  Multiply4 : Gain  Gain=em.noEM
  Product1 : Product
  Product2 : Product  Inputs=3
  Saturation : Saturate  UpperLimit=500  LowerLimit=-500
  Saturation1 : Saturate  UpperLimit=inf  LowerLimit=1
  Scope : Scope  NumInputPorts=6
  Speed-torrque characteristics : Lookup_n-D  NumberOfTableDimensions=1  BreakpointsForDimension1=em.speed  BeginIndexSearchUsingPreviousIndexResult=on  Table=em.trq  ExtrapMethod=Clip  UseLastTableValue=on  RndMeth=Simplest  InputSameDT=on
  Switch : Switch
  I_EM_current [A] : Outport  VectorParamsAs1DForOutWhenUnconnected=off
  M_EM [Nm] : Outport  Port=2  VectorParamsAs1DForOutWhenUnconnected=off
  tag scope: ETA_EM=global, I_EM_current=global, M_EM=global, M_EM_max=global, n_EM=global, u_EM=global
  wires:
  Speed-torrque characteristics/1 -> Multiply1/1, Product1/1  "M_EM_max"
  u_EM/1 -> Product1/2, [u_EM]
  U_Bat [V]/1 -> Memory/1  "U_Bat"
  Machine current demand/1(I_target [A]) -> Scope/1, Saturation/1  "I_target [A]"
  Saturation/1 -> Machine torque demand/2(I_current [A]), Scope/2  "I_current[A]"
  Machine torque demand/1(M_EM [Nm]) -> Switch/2, Multiply3/1, Scope/4, Product2/3, Abs/1  "M_EM [Nm]"
  Gain/1 -> Product2/2
  Divide/1 -> Scope/6, Multiply4/1  "I_EM_current"
  Math Function/1 -> Switch/1
  Electric machine efficiency mapping/1 -> Switch/3, Math Function/1  "Eta_EM"
  Switch/1 -> Product2/1
  Product2/1 -> Divide/1
  Abs/1 -> Electric machine efficiency mapping/1
  n_EM [rpm]/1 -> Electric machine efficiency mapping2/2, Scope/5, Saturation1/1, Electric machine efficiency mapping/2, Machine torque demand/1(n_EM [rpm]), Machine current demand/1("n_EM "), [n_EM], Speed-torrque characteristics/1  "n_EM [U/min]"
  Abs1/1 -> Electric machine efficiency mapping2/1
  Electric machine efficiency mapping2/1 -> Machine current demand/3(Eff_EM), [ETA_EM], Machine torque demand/3(Eff_EM)  "ETA_EM"
  Saturation1/1 -> Gain/1
  Memory/1 -> Machine torque demand/4(U_Bat [V]), Scope/3, Divide/2, Machine current demand/4(U_Bat [V])  "U_Bat [V]"
  Product1/1 -> Machine current demand/2(M_EM_target [Nm]), Abs1/1  "M_EM_target"
  Multiply4/1 -> I_EM_current [A]/1, [I_EM_current]
  Multiply3/1 -> M_EM [Nm]/1, [M_EM]
  Multiply1/1 -> [M_EM_max]

== system HDVSim_BEV_Truck/Hybrid ==
  note: Battery energy
  note: Regenerative braking energy
  Abs : Abs
  Abs1 : Abs
  Constant1 : Constant  Value=0
  Display1 : Display
  Display5 : Display
  Display6 : Display
  Gain1 : Gain  Gain=1/3600000
  Gain6 : Gain  Gain=1/3600000
  Gain7 : Gain  Gain=1/3600000
  Integrator1 : Integrator
  Integrator5 : Integrator
  Integrator6 : Integrator
  Out_Bat : Scope  NumInputPorts=4
  Product1 : Product
  Product3 : Product
  Scope1 : Scope
  Scope3 : Scope
  Scope7 : Scope  NumInputPorts=2
  Switch1 : Switch  Threshold=1
  wires:
  Product1/1 -> Switch1/1, Integrator6/1
  Gain1/1 -> Scope7/1, Display1/1  "E_REKUP_ES_AN [kWh]"
  Constant1/1 -> Switch1/3
  Integrator1/1 -> Gain1/1
  Switch1/1 -> Integrator1/1
  [REKUP] -> Scope7/2, Switch1/2  "REKUP"
  [U_Bat] -> Product1/2
  [I_current_BAT] -> Product1/1
  Gain7/1 -> Display6/1, Scope1/1
  Integrator6/1 -> Gain7/1
  [U_Bat] -> Abs1/1
  [I_current_BAT] -> Abs/1
  Product3/1 -> Integrator5/1
  Integrator5/1 -> Gain6/1
  Abs/1 -> Product3/1
  Abs1/1 -> Product3/2
  [SOC] -> Out_Bat/1  "SOC"
  [s_current1] -> Out_Bat/2  "s_current"
  [C_Rate] -> Out_Bat/3  "C_Rate"
  [I_EM_current] -> Out_Bat/4  "I_current"
  Gain6/1 -> Scope3/1, Display5/1  "Battery consumption [kWh]"

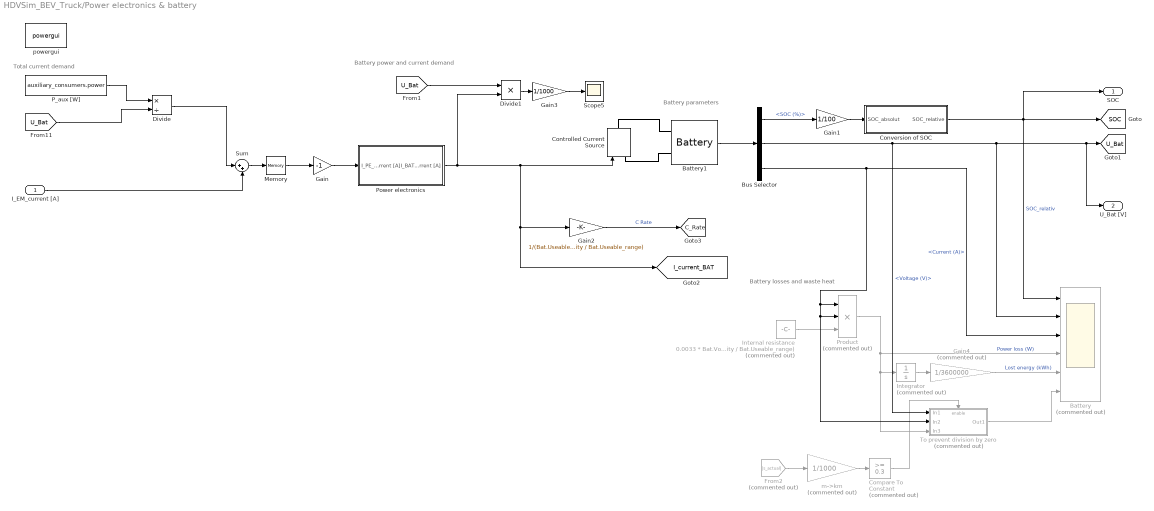
== system HDVSim_BEV_Truck/Power electronics & battery ==
  note: Battery parameters
  note: Battery power and current demand
  note: Total current demand
  note: Battery losses and waste heat
  I_EM_current [A] : Inport
  Battery : Scope  Commented=on  NumInputPorts=6
  Battery1 : electricdrivelib/Extra Sources/Battery  BatType=Lithium-Ion  ShowTempParam=off  ThermalPreset=no  ShowAgeParam=off  NomV=Bat.Voltage  NomQ=Bat.Useable_capacity / Bat.Useable_range  SOC=(Bat.SOC_start *Bat.Useable_range+(0.5-Bat.Useable_range/2))* 100  Batt_Tr=30  PresetModel=off  MaxQ=Bat.Useable_capacity / Bat.Useable_range *8077/7500  MinV=487.5  FullV=Bat.Voltage * 1.178  Dis_rate=0.2 * Bat.Useable_capacity / Bat.Useable_range  R=0.01 * Bat.Voltage / (Bat.Useable_capacity / Bat.Useable_range)  Normal_OP=Bat.Useable_capacity / Bat.Useable_range * 0.962  expZone="[Bat.Voltage*4339/4000     Bat.Useable_capacity / Bat.Useable_range/5]"  current=[5 25 50 250]  Units=Ampere-hour  Tci=20  NomT=20  T2=-30  MaxQ2=4.8  FullV2=7.1  Normal_OP2=5.72  expZone2="[6.58  1]"  Rca=0.6  ti=1000  Dp=0  Neq0=0  Tsim=1e6  Ta1=25  Qeol=5.4*0.9  Reol=0.013333*1.2  Char_age=[2.3478, 3]  Dis_age=[2.3478, 10]  N1=1500  N2=10500  N3=1000  N4=1400  Ta2=45  N5=950
      settings: SourceProductName=Simscape Electrical
  Bus Selector : BusSelector  OutputSignals=SOC (%),Voltage (V),Current (A)
  Compare To Constant : simulink/Logic and Bit Operations/Compare To Constant  Commented=on  relop=>=  const=0.3  OutDataTypeStr=uint8  ZeroCross=off
  Controlled Current Source : powerlib/Electrical Sources/Controlled Current Source  Initialize=off  Source_Type=DC  Amplitude=0  Phase=0  Frequency=0  Measurements=None
      settings: SourceProductName=Simscape Electrical
  Conversion of SOC : Subsystem
  Divide : Product  Inputs=*/
  Divide1 : Product  Inputs=**
  From2 : From  Commented=on  GotoTag=s_actual  TagVisibility=global
      settings: CloseFcn=tagdialog Close
  Gain : Gain  Gain=-1
  Gain1 : Gain  Gain=1/100
  Gain2 : Gain  Gain=1/(Bat.Useable_capacity / Bat.Useable_range)
  Gain3 : Gain  Gain=1/1000
  Gain4 : Gain  Commented=on  Gain=1/3600000
  Integrator : Integrator  Commented=on
  Internal resistance : Constant  Commented=on  Value=0.0033 * Bat.Voltage / (Bat.Useable_capacity / Bat.Useable_range)
  Memory : Memory
  P_aux [W] : Constant  Value=auxiliary_consumers.power
  Power electronics : Subsystem
  Product : Product  Commented=on  Inputs=3
  Scope5 : Scope
  Sum : Sum  Inputs=|++
  To prevent division by zero : Subsystem  Commented=on
  m->km : Gain  Commented=on  Gain=1/1000
  powergui : powerlib/powergui  Priority=1  SimulationMode=Discrete  SampleTime=sample_time  frequency=60  Iterations=50  frequencyindice=0  Pbase=100e6  ErrMax=1e-4  UnitsV=kV  UnitsW=MW  buscounter=0  FunctionMessages=on  echomessages=off  EnableUseOfTLC=off  CurrentSourceSwitches=off  DisableSnubberDevices=off  DisableRonSwitches=off  DisableVfSwitches=off  DisplayEquations=off  AutomaticDiscreteSolvers=off  SolverType=Tustin  Interpol=off  ExternalGateDelay=off  methode=off  Ts=100  x0status=blocks  SPID=off  SwTol=0  HookPort=off  NonlinearTolerance=1e-4  nMaxIteration=100  ContinueOnMaxIteration=off  RestoreLinks=warning  ResistiveCurrentMeasurement=off  Frange=[0:2:500]  Ylog=off  Xlog=on  ShowGrid=off  save=off  variable=ZData  structure=0  ZoomFFT=off  StartTime=0.0  cycles=1  DisplayStyle=1  fundamental=60  FreqAxis=off  MaxFrequency=1000  frequencyindicesteady=1  RmsSteady=1  display=off
      settings: SourceProductName=Simscape Electrical
  SOC : Outport  VectorParamsAs1DForOutWhenUnconnected=off
  U_Bat [V] : Outport  Port=2  VectorParamsAs1DForOutWhenUnconnected=off
  tag scope: C_Rate=global, I_current_BAT=global, SOC=global, U_Bat=global
  wires:
  Battery1/1 -> Bus Selector/1
  Bus Selector/1 -> Gain1/1  "<SOC (%)>"
  Gain1/1 -> Conversion of SOC/1(SOC_absolut)
  Memory/1 -> Gain/1
  Gain/1 -> Power electronics/1(I_PE_current [A])
  Gain2/1 -> [C_Rate]  "C Rate"
  [U_Bat] -> Divide/2
  P_aux [W]/1 -> Divide/1
  Divide/1 -> Sum/1
  Sum/1 -> Memory/1
  I_EM_current [A]/1 -> Sum/2
  Power electronics/1(I_BAT_current [A]) -> Divide1/2, Controlled Current Source/1, [I_current_BAT], Gain2/1
  Conversion of SOC/1(SOC_relative) -> [SOC], SOC/1, Battery/1  "SOC_relativ"
  [U_Bat] -> Divide1/1
  Gain3/1 -> Scope5/1
  Divide1/1 -> Gain3/1
  m->km/1 -> Compare To Constant/1
  Compare To Constant/1 -> To prevent division by zero/Enable
  From2/1 -> m->km/1
  Gain4/1 -> Battery/5  "Lost energy (kWh)"
  To prevent division by zero/1(Out1) -> Battery/6
  Product/1 -> Battery/4, To prevent division by zero/3(In3), Integrator/1  "Power loss (W)"
  Internal resistance/1 -> Product/3
  Integrator/1 -> Gain4/1
  Bus Selector/3 -> To prevent division by zero/2(In2), Product/2, Product/1, Battery/3  "<Current (A)>"
  Bus Selector/2 -> To prevent division by zero/1(In1), Battery/2, U_Bat [V]/1, [U_Bat]  "<Voltage (V)>"
  connections:
  Battery1/LConn2 -- Controlled Current Source/LConn1
  Battery1/LConn1 -- Controlled Current Source/RConn1

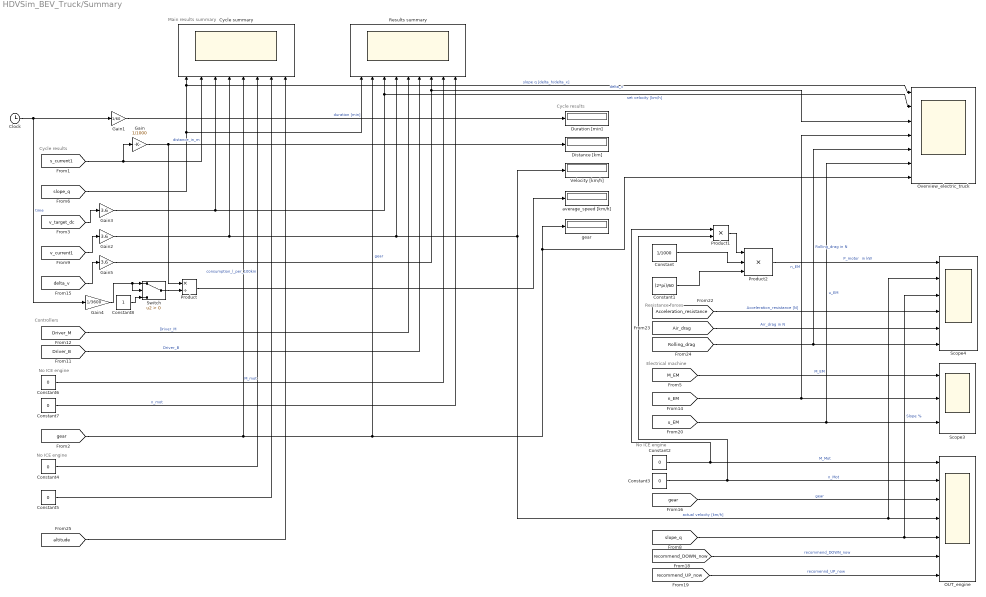
== system HDVSim_BEV_Truck/Summary ==
  note: Main results summary
  note: Cycle results
  note: Controllers
  note: Cycle results
  note: Resistance forces
  note: Electrical machine
  note: No ICE engine
  note: No ICE engine
  note: No ICE engine
  Clock : Clock
  Constant : Constant  Value=1/1000
  Constant1 : Constant  Value=(2*pi)/60
  Constant{2..7} (6 alike) : Constant  Value=0
  Constant8 : Constant
  Cycle summary : Scope  NumInputPorts=8
  Distance [km] : Display
  Duration [min] : Display
  Gain : Gain  Gain=1/1000
  Gain1 : Gain  Gain=1/60
  Gain2 : Gain  Gain=3.6
  Gain3 : Gain  Gain=3.6
  Gain4 : Gain  Gain=1/3600
  Gain5 : Gain  Gain=3.6
  OUT_engine : Scope  NumInputPorts=7
  Overview_electric_truck : Scope  NumInputPorts=7
  Product : Product  Inputs=*/  RndMeth=Zero
  Product1 : Product
  Product2 : Product  Inputs=3
  Results summary : Scope  NumInputPorts=9
  Scope3 : Scope  NumInputPorts=3
  Scope4 : Scope  NumInputPorts=6
  Switch : Switch  Criteria=u2 > Threshold
  Velocity [km/h] : Display
  average_speed [km/h] : Display
  gear : Display
  wires:
  [v_current1] -> Gain2/1
  [s_current1] -> Cycle summary/2, Gain/1  "distance_in_m"
  Gain/1 -> Distance [km]/1, Product/1
  Clock/1 -> Gain1/1, Gain4/1  "time"
  Gain1/1 -> Duration [min]/1  "duration [min]"
  Gain2/1 -> OUT_engine/4, Scope4/2, Velocity [km/h]/1, Results summary/4, Cycle summary/4  "actual velocity [km/h]"
  [gear] -> gear/1, Overview_electric_truck/7, Results summary/2, Cycle summary/5  "gear"
  [v_target_dc] -> Gain3/1
  [slope_q] -> Results summary/1, Overview_electric_truck/1, Cycle summary/1  "slope q [delta_h/delta_x]"
  Constant4/1 -> Cycle summary/6  "consumption_l_per_100km"
  Gain3/1 -> Results summary/3, Overview_electric_truck/2, Cycle summary/3  "set velocity [km/h]"
  Gain4/1 -> Switch/2, Switch/1
  Product/1 -> average_speed [km/h]/1
  Constant5/1 -> Cycle summary/7
  [Driver_M] -> Results summary/5  "Driver_M"
  [Driver_B] -> Results summary/6  "Driver_B"
  Constant6/1 -> Results summary/8  "M_mot"
  [delta_v] -> Gain5/1
  Constant2/1 -> OUT_engine/1, Product1/1  "M_Mot"
  Constant3/1 -> Product1/2, OUT_engine/2  "n_Mot"
  [gear] -> OUT_engine/3  "gear"
  [recommend_DOWN_now] -> OUT_engine/6  "recommend_DOWN_now"
  [recommend_UP_now] -> OUT_engine/7  "recomennd_UP_now"
  [slope_q] -> Scope4/3, OUT_engine/5  "Slope %"
  Gain5/1 -> Results summary/7, Overview_electric_truck/3  "delta_v"
  Constant7/1 -> Results summary/9  "n_mot"
  [M_EM] -> Scope3/1  "M_EM"
  [n_EM] -> Overview_electric_truck/4, Scope3/2  "n_EM"
  [u_EM] -> Overview_electric_truck/6, Scope3/3  "u_EM"
  Product1/1 -> Product2/1
  Constant/1 -> Product2/2
  Product2/1 -> Scope4/1  "P_motor  in kW"
  Constant1/1 -> Product2/3
  [Acceleration_resistance] -> Scope4/4  "Acceleration_resistance [N]"
  [Air_drag] -> Scope4/5  "Air_drag in N"
  [Rolling_drag] -> Overview_electric_truck/5, Scope4/6  "Rolling_drag in N"
  Switch/1 -> Product/2
  Constant8/1 -> Switch/3
  [altitude] -> Cycle summary/8

== system HDVSim_BEV_Truck/Tires ==
  M_tire [Nm] : Inport
  v_current [m/s] : Inport  Port=2
  F=M/r : Product  Inputs=*/
  Tire radius : Constant  Value=tires.radius
  "phi. -> n[1/min]" : Gain  Gain=60/2/pi
  phi. = v/r : Product  Inputs=/*
  n_tire [rpm] : Outport  VectorParamsAs1DForOutWhenUnconnected=off
  F_x [N] : Outport  Port=2  VectorParamsAs1DForOutWhenUnconnected=off
  wires:
  phi. = v/r/1 -> "phi. -> n[1/min]"/1
  "phi. -> n[1/min]"/1 -> n_tire [rpm]/1
  Tire radius/1 -> phi. = v/r/1, F=M/r/2
  v_current [m/s]/1 -> phi. = v/r/2
  M_tire [Nm]/1 -> F=M/r/1
  F=M/r/1 -> F_x [N]/1

== system HDVSim_BEV_Truck/Transmission ==
  note: Transmission torque multiplication through the different gears
  M_EM [Nm] : Inport
  n_Gearbox [rpm] : Inport  Port=2
  v_target [m/s] : Inport  Port=3
  delta_v : Inport  Port=4
  Compare To Constant : simulink/Logic and Bit Operations/Compare To Constant  relop=~=  const=1  OutDataTypeStr=boolean
  Determine when shifting occurs : Subsystem  TreatAsAtomicUnit=on
  Memory1 : Memory
  Number of gears : Constant  Value=transmission.z  VectorParams1D=off
  Saturation : Saturate  UpperLimit=inf  LowerLimit=0
  Shifting rules : Stateflow chart  TreatAsAtomicUnit=on
  Slope-> angle : Trigonometry  Operator=atan
  Torque flow through the transmission : Subsystem
  Transmission gears : Constant  Value=transmission.z  VectorParams1D=off
  ZKU : Subsystem
  init_gear : Constant  Value=transmission.init_gear
  n_EM [rpm] : Outport  VectorParamsAs1DForOutWhenUnconnected=off
  M_Gearbox [Nm] : Outport  Port=2  VectorParamsAs1DForOutWhenUnconnected=off
  tag scope: gear=global, i_gearbox=global, recommend_DOWN_now=global, recommend_UP_now=global
  wires:
  n_Gearbox [rpm]/1 -> Torque flow through the transmission/2(n_gearbox_out [1/min]), Determine when shifting occurs/3(n_Getr_out [1/min])
  Torque flow through the transmission/2(M_gearbox_out [Nm]) -> [M_Getr_out], M_Gearbox [Nm]/1
  Torque flow through the transmission/1(n_gearbox_in [1/min]) -> Saturation/1
  init_gear/1 -> Shifting rules/1(init_gear)
  Determine when shifting occurs/27(check_torque_reseve_2lower) -> Shifting rules/29(check_torque_reserve_2lower)
  Determine when shifting occurs/26(check_torque_reseve_2higher) -> Shifting rules/28(check_torque_reserve_2higher)
  Determine when shifting occurs/1(reccommend_down_2higher) -> Shifting rules/3(recommend_down_2higher)
  Determine when shifting occurs/2(reccommend_down_1higher) -> Shifting rules/4(recommend_down_1higher)
  Determine when shifting occurs/3(reccommend_down_now) -> Shifting rules/5(recommend_down_now), [recommend_DOWN_now]
  Determine when shifting occurs/4(reccommend_down_1lower) -> Shifting rules/6(recommend_down_1lower)
  Determine when shifting occurs/5(reccommend_down_2lower) -> Shifting rules/7(recommend_down_2llower)
  Determine when shifting occurs/6(reccommend_up_2higher) -> Shifting rules/8(recommend_up_2higher)
  Determine when shifting occurs/7(reccommend_up_1higher) -> Shifting rules/9(recommend_up_1higher)
  Determine when shifting occurs/8(reccommend_up_now) -> Shifting rules/10(recommend_up_now), [recommend_UP_now]
  Determine when shifting occurs/9(reccommend_up_1lower) -> Shifting rules/11(recommend_up_1lower)
  Determine when shifting occurs/10(reccommend_up_2lower) -> Shifting rules/12(recommend_up_2lower)
  Determine when shifting occurs/11(check_n_min_2higher) -> Shifting rules/13(check_n_min_2higher)
  Determine when shifting occurs/12(check_n_min_1higher) -> Shifting rules/14(check_n_min_1higher)
  Determine when shifting occurs/13(check_n_min_now) -> Shifting rules/15(check_n_min_now)
  Determine when shifting occurs/14(check_n_min_1lower) -> Shifting rules/16(check_n_min_1lower)
  Determine when shifting occurs/15(check_n_min_2lower) -> Shifting rules/17(check_n_min_2lower)
  Determine when shifting occurs/16(check_n_max_2higher) -> Shifting rules/18(check_n_max_2higher)
  Determine when shifting occurs/17(check_n_max_1higher) -> Shifting rules/19(check_n_max_1higher)
  Determine when shifting occurs/18(check_n_max_now) -> Shifting rules/20(check_n_max_now)
  Determine when shifting occurs/19(check_n_max_1lower) -> Shifting rules/21(check_n_max_1lower)
  Determine when shifting occurs/20(check_n_max_2lower) -> Shifting rules/22(check_n_max_2lower)
  Determine when shifting occurs/21(check_M_max_2higher) -> Shifting rules/23(check_M_max_2higher)  "check_M_max_2higher"
  Determine when shifting occurs/22(check_M_max_1higher) -> Shifting rules/24(check_M_max_1higher)  "check_M_max_1higher"
  Determine when shifting occurs/23(check_M_max_now) -> Shifting rules/25(check_M_max_now)  "check_M_max_now"
  Determine when shifting occurs/24(check_M_max_1lower) -> Shifting rules/26(check_M_max_1lower)  "check_M_max_1lower"
  Determine when shifting occurs/25(check_M_max_2lower) -> Shifting rules/27(check_M_max_2lower)  "check_M_max_2lower"
  Memory1/1 -> [gear], [Gear], ZKU/1(Gear), Torque flow through the transmission/3(Gear)
  M_EM [Nm]/1 -> Torque flow through the transmission/1(M_gearbox_in [Nm])  "M_gearbox_in [Nm]"
  Saturation/1 -> n_EM [rpm]/1
  Torque flow through the transmission/3(i_gearbox) -> [i_gearbox]
  delta_v/1 -> Determine when shifting occurs/4(delta_v)
  v_target [m/s]/1 -> Determine when shifting occurs/5(v_target [m/s])
  Number of gears/1 -> Shifting rules/2(z)
  Transmission gears/1 -> Compare To Constant/1
  Compare To Constant/1 -> Determine when shifting occurs/Enable
  [slope_q] -> Slope-> angle/1
  Slope-> angle/1 -> Determine when shifting occurs/6(alpha)
  [gear] -> Memory1/1
  Shifting rules/1(gear) -> [gear]
  [M_Getr_out] -> Determine when shifting occurs/2(M_Getr_out [Nm])
  [Gear] -> Determine when shifting occurs/1(Gear)

== system HDVSim_BEV_Truck/Vehicle ==
  note: Net tractive force applied on the vehicle
  note: Vehicle acceleration
  F_x [N] : Inport
  u_KB : Inport  Port=2
  alpha [rad] : Inport  Port=3
  Add : Sum  Inputs=-+-
  Braking force [N] : Product  RndMeth=Zero
  Cargo weight : Constant  Value=vehicle.payload
  Driving resistances without acceleration : Subsystem
  F_brake_max : Constant  Value=vehicle.F_brake_max
  Integrator : Integrator
  Integrator1 : Integrator  InitialCondition=cycle.speed_init  LimitOutput=on  LowerSaturationLimit=0
  Product : Product  Inputs=3
  Product2 : Product  Inputs=*/  RndMeth=Zero
  Product3 : Product  Inputs=**  RndMeth=Zero
  Sum1 : Sum  Inputs=|++
  Sum2 : Sum  Inputs=|++
  Vehicle weight : Constant  Value=vehicle.mass
  v_current [m/s] : Outport  VectorParamsAs1DForOutWhenUnconnected=off
  s_current [m] : Outport  Port=2  VectorParamsAs1DForOutWhenUnconnected=off
  tag scope: Acceleration_resistance=global, s_current1=global, v_current1=global
  wires:
  alpha [rad]/1 -> Driving resistances without acceleration/1(alpha [rad])
  Add/1 -> Product2/1
  Driving resistances without acceleration/1(F_W [N]) -> Add/3
  F_x [N]/1 -> Add/2  "F_x"
  F_brake_max/1 -> Braking force [N]/2
  Integrator/1 -> [s_current1], s_current [m]/1  "s_current"
  Cargo weight/1 -> Sum1/2, Sum2/2
  Sum1/1 -> Product2/2
  Vehicle weight/1 -> Sum2/1, Product3/2
  Product3/1 -> Sum1/1
  Integrator1/1 -> Driving resistances without acceleration/2(v [m/s]), v_current [m/s]/1, [v_current1], Integrator/1  "v_current"
  [lamda] -> Product/1, Product3/1
  u_KB/1 -> Braking force [N]/1
  Braking force [N]/1 -> Add/1  "F_brake"
  Product2/1 -> Integrator1/1, Product/3  "a"
  Product/1 -> [Acceleration_resistance]
  Sum2/1 -> Product/2  "m_total"

== system HDVSim_BEV_Truck/Active cruise control1/Braking from upper speed limit ==
  v_target [m/s] : Inport
  Add3 : Sum  Inputs=+-
  Constant1 : Constant  Value=90/3.6
  Constant10 : Constant  Value=prospective_cruise_control
  Constant6 : Constant  Value=v_PPC_delta
  Constant7 : Constant  Value=0
  Constant8 : Constant  Value=0
  Saturation Dynamic : simulink/Discontinuities/Saturation Dynamic  OutMin=[]  OutMax=[]  OutDataTypeStr=Inherit: Same as second input  OutDataType=fixdt(1, 16)  OutScaling=2^-10  DoSatur=off
  Switch3 : Switch  Criteria=u2 > Threshold
  Out1 : Outport  VectorParamsAs1DForOutWhenUnconnected=off
  wires:
  Switch3/1 -> Out1/1
  Constant6/1 -> Saturation Dynamic/2
  Constant1/1 -> Add3/1
  Constant7/1 -> Switch3/3
  Add3/1 -> Saturation Dynamic/1
  Constant8/1 -> Saturation Dynamic/3
  Constant10/1 -> Switch3/2
  v_target [m/s]/1 -> Add3/2
  Saturation Dynamic/1 -> Switch3/1
